simulink model "Ejemplo_01_simulink_comparacion"  (R2018a)
settings: Solver=VariableStepAuto  StartTime=0.0  StopTime=10.0  RelTol=1e-3
settings Model: Creator=LENOVO  LastModifiedBy=LENOVO

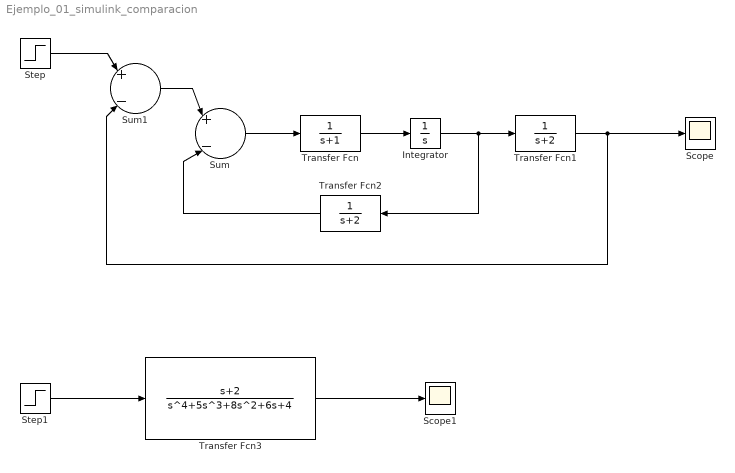
== system Ejemplo_01_simulink_comparacion ==
  Integrator : Integrator
  Scope : Scope
  Scope1 : Scope
  Step : Step  SampleTime=0
  Step1 : Step  SampleTime=0
  Sum : Sum  Inputs=|+|-|
  Sum1 : Sum  Inputs=|+|-|
  Transfer Fcn : TransferFcn  Denominator=[1 1]
  Transfer Fcn1 : TransferFcn  Denominator=[1 2]
  Transfer Fcn2 : TransferFcn  Denominator=[1 2]
  Transfer Fcn3 : TransferFcn  Numerator=[1 2]  Denominator=[1 5 8 6 4]
  wires:
  Sum/1 -> Transfer Fcn/1
  Transfer Fcn/1 -> Integrator/1
  Integrator/1 -> Transfer Fcn2/1, Transfer Fcn1/1
  Sum1/1 -> Sum/1
  Transfer Fcn2/1 -> Sum/2
  Transfer Fcn1/1 -> Scope/1, Sum1/2
  Step/1 -> Sum1/1
  Step1/1 -> Transfer Fcn3/1
  Transfer Fcn3/1 -> Scope1/1
